simulink subsystem "ReLU_layer"  (R2021b)
settings: Solver=VariableStepAuto  StartTime=0.0  StopTime=10.0  RelTol=1e-3
settings Model: Creator=bogru  LastModifiedBy=bogru

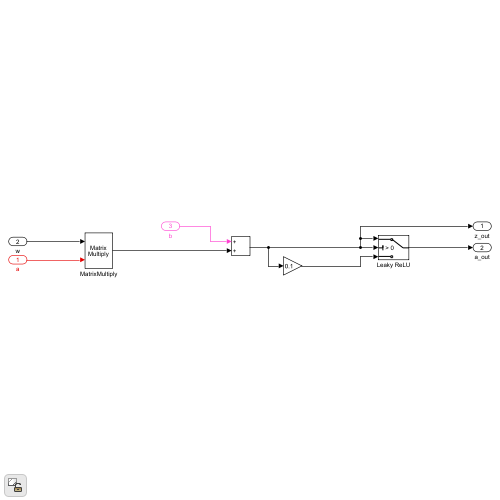
[thumbnail: Simulink's stored preview of the top-level diagram]
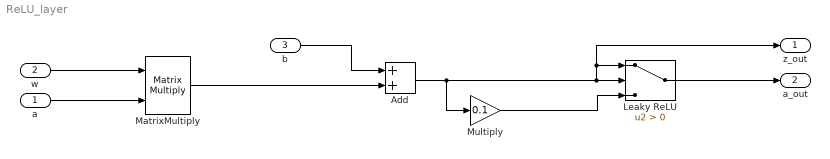
== system ReLU_layer ==
  a : Inport  SampleTime=1
  w : Inport  Port=2  SampleTime=1
  b : Inport  Port=3  SampleTime=1
  Add : Sum  AccumDataTypeStr=fixdt(1,18,12)
  Leaky ReLU : Switch  Criteria=u2 > Threshold
  MatrixMultiply : Product  Multiplication=Matrix(*)  OutDataTypeStr=fixdt(1,18,12)
  Multiply : Gain  Gain=0.1
  z_out : Outport  OutDataTypeStr=fixdt(1,18,12)
  a_out : Outport  Port=2  OutDataTypeStr=fixdt(1,18,12)
  wires:
  b/1 -> Add/1
  MatrixMultiply/1 -> Add/2
  Add/1 -> z_out/1, Leaky ReLU/1, Leaky ReLU/2, Multiply/1
  a/1 -> MatrixMultiply/2
  Multiply/1 -> Leaky ReLU/3
  w/1 -> MatrixMultiply/1
  Leaky ReLU/1 -> a_out/1
